simulink model "Laengsdynamikmodell_NEmo_MonteCarlo"  (R2019b)
settings: Solver=FixedStepAuto  StartTime=0.0  StopTime=1  FixedStep=SampleTime  RelTol=1e-3
undefined symbols (not defined in the file): C_RR, DiscIntNeverNeededParam, gravity, OM_PEl_M_Map, omega_Mot, PEl_MotVector, power_map_Mot, r_dyn, torque_Mot, UncertaintyMappedLosses, UncertaintyRollerDynamometer, UncertaintyTabledConsumption, VehMass
libraries: Driver_PI x1, Longitudinal_DrivingCycles x1, Acceleration_Calculation x1, Air_Resistance x1, Roll_Resistance x1, Slope_Resistance x1, Simple_Auxiliary x1, Gear_Stage x1, DCAC_Converter x1
(part 1 of 2)
settings Model: SimulationMode=accelerator  NumberOfSteps=1000  OrderedModelArguments=off  Creator=Tony  LastModifiedBy=ga69qig
settings DataIOCC: ReturnWorkspaceOutputs=off
settings DebuggingCC: ArithmeticOperatorsInVariantConditions=warning
settings SFSimCC: SimUseLocalCustomCode=off  CustomCodeUndefinedFunction=UseInterfaceOnly
settings RTWCC: RTWUseLocalCustomCode=off
settings CodeAppCC: StateflowObjectComments=on

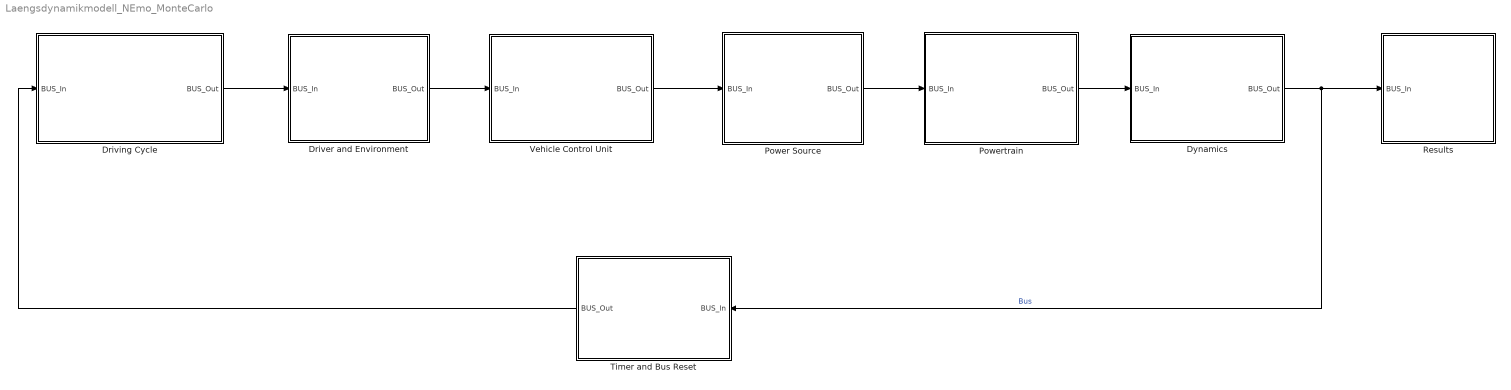
== system Laengsdynamikmodell_NEmo_MonteCarlo ==
  Driver and Environment : Subsystem
      mask help:
      | <Author> Alexander Koch based on Stefan Müller, Stephan Rohr
      | <Date> 03/04/2017
      |
      | <Description>
      | Consist of a Bus In and a Bus Out Block. To Select Signals from the Bus open the Bus In Block, to write signals to the Bus under a certain tab name open the bus out block. For further information, please read the discription of the Bus In and Bus out Block
      |
      | The Block automaticlly disconnects the link to the library block after opening the first time
      |
      | <Parameters>
      | -
      |
      | <Inputs>
      | BUS_In [Bus]
      |
      | <Outputs>
      | Bus_Out [Bus]
      settings: OpenFcn=|
      | set_param(gcb(),'LinkStatus','none')
      | open_system(gcb(),'force')
      mask Display:
      | [picturexpos,pictureypos,picturewidth,pictureheight] = ...
      |     CalcBlockPicturePosition(gcb,1,0.01,0.1,30,30); % calculating picture position depending on Block size and minimum margin size
      | image('Driver_PI.svg',[picturexpos pictureypos picturewidth pictureheight]); % plot picture to block
  Driving Cycle : Subsystem
      mask help:
      | <Author> Alexander Koch based on Stefan Müller, Stephan Rohr
      | <Date> 03/04/2017
      |
      | <Description>
      | Consist of a Bus In and a Bus Out Block. To Select Signals from the Bus open the Bus In Block, to write signals to the Bus under a certain tab name open the bus out block. For further information, please read the discription of the Bus In and Bus out Block
      |
      | The Block automaticlly disconnects the link to the library block after opening the first time
      |
      | <Parameters>
      | -
      |
      | <Inputs>
      | BUS_In [Bus]
      |
      | <Outputs>
      | Bus_Out [Bus]
      settings: OpenFcn=|
      | set_param(gcb(),'LinkStatus','none')
      | open_system(gcb(),'force')
      mask Display:
      | [picturexpos,pictureypos,picturewidth,pictureheight] = ...
      |     CalcBlockPicturePosition(gcb,1,0.01,0.1,50,50); % calculating picture position depending on Block size and minimum margin size
      | image('Longitudinal_DrivingCycles.svg',[picturexpos pictureypos picturewidth pictureheight]); % plot picture to block
  Dynamics : Subsystem
      mask help:
      | <Author> Alexander Koch based on Stefan Müller, Stephan Rohr
      | <Date> 03/04/2017
      |
      | <Description>
      | Consist of a Bus In and a Bus Out Block. To Select Signals from the Bus open the Bus In Block, to write signals to the Bus under a certain tab name open the bus out block. For further information, please read the discription of the Bus In and Bus out Block
      |
      | The Block automaticlly disconnects the link to the library block after opening the first time
      |
      | <Parameters>
      | -
      |
      | <Inputs>
      | BUS_In [Bus]
      |
      | <Outputs>
      | Bus_Out [Bus]
      settings: OpenFcn=|
      | set_param(gcb(),'LinkStatus','none')
      | open_system(gcb(),'force')
      mask Display:
      | [picturexpos,pictureypos,picturewidth,pictureheight] = ...
      |     CalcBlockPicturePosition(gcb,1,0.01,0.1,40,50); % calculating picture position depending on Block size and minimum margin size
      | image('Acceleration_Calculation.svg',[picturexpos pictureypos picturewidth pictureheight]); % plot picture to block
  Power Source : Subsystem
      mask help:
      | <Author> Alexander Koch based on Stefan Müller, Stephan Rohr
      | <Date> 03/04/2017
      |
      | <Description>
      | Consist of a Bus In and a Bus Out Block. To Select Signals from the Bus open the Bus In Block, to write signals to the Bus under a certain tab name open the bus out block. For further information, please read the discription of the Bus In and Bus out Block
      |
      | The Block automaticlly disconnects the link to the library block after opening the first time
      |
      | <Parameters>
      | -
      |
      | <Inputs>
      | BUS_In [Bus]
      |
      | <Outputs>
      | Bus_Out [Bus]
      settings: OpenFcn=|
      | set_param(gcb(),'LinkStatus','none')
      | open_system(gcb(),'force')
      mask Display:
      | [picturexpos,pictureypos,picturewidth,pictureheight] = ...
      |     CalcBlockPicturePosition(gcb,3/6,0.01,0.1,40,40); % calculating picture position depending on Block size and minimum margin size
      | image('Constant_Power_Source.svg',[picturexpos pictureypos picturewidth pictureheight]); % plot picture to block
  Powertrain : Subsystem
      mask help:
      | <Author> Alexander Koch based on Stefan Müller, Stephan Rohr
      | <Date> 03/04/2017
      |
      | <Description>
      | Consist of a Bus In and a Bus Out Block. To Select Signals from the Bus open the Bus In Block, to write signals to the Bus under a certain tab name open the bus out block. For further information, please read the discription of the Bus In and Bus out Block
      |
      | The Block automaticlly disconnects the link to the library block after opening the first time
      |
      | <Parameters>
      | -
      |
      | <Inputs>
      | BUS_In [Bus]
      |
      | <Outputs>
      | Bus_Out [Bus]
      settings: OpenFcn=|
      | set_param(gcb(),'LinkStatus','none')
      | open_system(gcb(),'force')
      mask Display:
      | [picturexpos,pictureypos,picturewidth,pictureheight] = ...
      |     CalcBlockPicturePosition(gcb,1,0.01,0.1,40,40); % calculating picture position depending on Block size and minimum margin size
      | image('Electric_Drive_Simple_Efficiency.svg',[picturexpos pictureypos picturewidth pictureheight]); % plot picture to block
  Results : Subsystem
      mask help:
      | <Author> Alexander Koch
      | <Date> 03/04/2017
      | <Predecessor> Stefan Müller, Stephan Rohr
      |
      | <Description>
      | Consist of a Bus In and a Bus Out Block. To Select Signals from the Bus open the Bus In Block, to write signals to the Bus under a certain tab name open the bus out block. For further information, please read the discription of the Bus In and Bus out Block
      |
      | The Block automaticlly disconnects the link to the library block after opening the first time
      |
      | <Parameters>
      | -
      |
      | <Inputs>
      | Bus [Bus]
      |
      | <Outputs>
      | Bus [Bus]
      settings: OpenFcn=|
      | set_param(gcb(),'LinkStatus','none')
      | open_system(gcb(),'force')
      mask Display:
      | [picturexpos,pictureypos,picturewidth,pictureheight] = ...
      |     CalcBlockPicturePosition(gcb,1,0.01,0.1,40,10); % calculating picture position depending on Block size and minimum margin size
      | image('Scopes_Simulation.svg',[picturexpos pictureypos picturewidth pictureheight]); % plot picture to block
  Timer and Bus Reset : Subsystem
      settings: OpenFcn=|
      | set_param(gcb(),'LinkStatus','none')
      | open_system(gcb(),'mask')
      mask DialogControl RefreshBus Prompt: Refresh Bus
      mask DialogControl RefreshBus Callback: TimerandBusResetRefreshBus()
      mask Display:
      | [picturexpos,pictureypos,picturewidth,pictureheight] = ...
      |     CalcBlockPicturePosition(gcb,1,0.01,0.1,50,50); % calculating picture position depending on Block size and minimum margin size
      | image('reset.png',[picturexpos pictureypos picturewidth pictureheight]); % plot picture to block
  Vehicle Control Unit : Subsystem
      mask help:
      | <Author> Alexander Koch based on Stefan Müller, Stephan Rohr
      | <Date> 03/04/2017
      |
      | <Description>
      | Consist of a Bus In and a Bus Out Block. To Select Signals from the Bus open the Bus In Block, to write signals to the Bus under a certain tab name open the bus out block. For further information, please read the discription of the Bus In and Bus out Block
      |
      | The Block automaticlly disconnects the link to the library block after opening the first time
      |
      | <Parameters>
      | -
      |
      | <Inputs>
      | BUS_In [Bus]
      |
      | <Outputs>
      | Bus_Out [Bus]
      settings: OpenFcn=|
      | set_param(gcb(),'LinkStatus','none')
      | open_system(gcb(),'force')
      mask Display:
      | [picturexpos,pictureypos,picturewidth,pictureheight] = ...
      |     CalcBlockPicturePosition(gcb,1,0.01,0.1,30,30); % calculating picture position depending on Block size and minimum margin size
      | image('Control_Unit_Simple.svg',[picturexpos pictureypos picturewidth pictureheight]); % plot picture to block
  wires:
  Power Source/1(BUS_Out) -> Powertrain/1(BUS_In)
  Driver and Environment/1(BUS_Out) -> Vehicle Control Unit/1(BUS_In)
  Driving Cycle/1(BUS_Out) -> Driver and Environment/1(BUS_In)
  Vehicle Control Unit/1(BUS_Out) -> Power Source/1(BUS_In)
  Timer and Bus Reset/1(BUS_Out) -> Driving Cycle/1(BUS_In)
  Dynamics/1(BUS_Out) -> Timer and Bus Reset/1(BUS_In), Results/1(BUS_In)  "Bus"
  Powertrain/1(BUS_Out) -> Dynamics/1(BUS_In)

== system Laengsdynamikmodell_NEmo_MonteCarlo/Driver and Environment ==
  BUS_In : Inport
  BUS IN : Subsystem
      mask help:
      | <Author> Alexander Koch based on Stefan Müller, Stephan Rohr
      | <Date> 02/05/2017
      |
      | <Description>
      | Automated BUS IN Block for the Bus System. After the Bus In is connected and receives signals it is possible to choose the required signals by clicking on the block. After choosing the signals it is possible to push the Refresh button. This button builds the required amount of outputs, connects the Bus Selector and the Outputs and rename all the outputs with the corresponding signal name.
      |
      | The Block automaticlly disconnects the link to the library block after opening the first time
      |
      | <Parameters>
      | -
      |
      | <Inputs>
      | Bus [Bus]
      |
      | <Outputs>
      | Bus [Bus]
      | SignalName[-]
      mask init:
      | BusInInitFct()
      settings: OpenFcn=|
      | set_param(gcb(),'LinkStatus','none')
      | open_system(gcb(),'mask')
      | open_system(strcat(gcb(),'/Bus Selector'),'Parameter')
      mask DialogControl ParameterGroupVar Prompt: Refresh
      mask DialogControl RefreshOutputs Prompt: Refresh all Output Names
      mask DialogControl RefreshOutputs Callback: BusInInitFct()
  BUS OUT : Subsystem  mask{NumberofInputs=6, NameSys='Driver and Enironment'}
      mask prompts: NumberofInputs "Numper of costum inputs"; NameSys "Name of Bus Subsystem"
      mask help:
      | <Author> Alexander Koch based on Stefan Müller, Stephan Rohr
      | <Date> 02/05/2017
      |
      | <Description>
      | Automated BUS Out Block for the Bus System. Allows to enter the Number of costum inputs and the name of the bus system. After entering the parameters the required amout of Inputs are built and connected to the Bus Creator. The signal names that are connected to the inputs In1, ..., InN are automatically adopted at the Bus signal names and can be found in the Bus under the name of the Bus Subsystem. If the signal (line) to the Inport has no name, the name of the previous blocks outport is taken. If this is not possible, the name if the previous block is taken for the Bus signal name.
      |
      | Additional, there are two buttons. The Refresh Input Names refreshes all Input Names. This is required if signal names are changed or signals are connected for the first time. To build a new system or if another Subsystem is added between existing subsystems, the Refresh Bus Selector is required at every subsystem that is calculated after the new subsystem.
      |
      | The Block automaticlly disconnects the link to the library block after opening the first time
      |
      | <Parameters>
      | Number of costum inputs [-]
      | Name of Bus Subsystem ['abc']
      |
      | <Inputs>
      | Bus [Bus]
      | In1 [ ]
      |
      | <Outputs>
      | Bus [Bus]
      mask init:
      | BusRefreshInputs()
      settings: OpenFcn=|
      | set_param(gcb(),'LinkStatus','none')
      | open_system(gcb(),'mask')
      mask DialogControl Container3 Prompt: Refresh
      mask DialogControl RefreshInputNames Prompt: Refresh Input Names
      mask DialogControl RefreshInputNames Callback: BusRefreshLineNames()
      mask DialogControl RefreshBusSelector Prompt: Refresh Bus Selector
      mask DialogControl RefreshBusSelector Callback: BusRefreshBusSelector()
  Constant Environment : Subsystem  AncestorBlock=Constant_Environment/Constant Environment  mask(SB){Ground_Slope=0, Long_Wind_Speed=0, Ambient_P=101325, Ambient_Temp=293.15, LocalSampleTime=-1}
      mask prompts: Ground_Slope "Ground Slope [rad]"; Long_Wind_Speed "Longitudinal Wind Velocity [m/s]"; Ambient_P "Ambient Pressure [Pa]"; Ambient_Temp "Ambient Temperature [K]"; LocalSampleTime "Local System Sample-Time [s]"
      mask help:
      | <Author> Tony Weiss based on Alexander Koch </Author>
      | <Date> 31/12/2017 </Date>
      | <Source>
      | [1] A. Koch, “Aufbau einer modularen Komponentenbibliothek für Gesamtfahrzeugsimulationen in Matlab/Simulink,” Technische Universität München, München, 2017
      | </Source>
      |
      | <Description>
      | Requires a ground slope, a longitudinal wind velocity, an ambient temperature and an ambient pressure and gives these constant values as signals. Ambient pressure is preset to 101325 Pa (standard pressure at sea level), ambient temperature is preset to 298.15 K.
      | </Description>
      mask init:
      | GlobalSampleTime = CalcGlobalSampleTime(LocalSampleTime);
      mask Help:
      | <Parameters>
      | Ground Slope [rad]
      | Longitudinal Wind Velocity [m/s]
      | Ambient Temperature [K]
      | Ambient Pressure [Pa]
      | Local System Sample-Time [s]
      | 	<Min> GlobalSampleTime </Min>
      | Global Sample-Time [s]
      | </Parameters>
      | 
      | <Inputs>
      | </Inputs>
      | 
      | <Outputs>
      | GroundSlope [rad]
      | LongWindVelocity [m/s]
      | AmbientTemperature [K]
      | AmbientPressure [Pa]
      | </Outputs>
      mask TypeOptions Ground_Slope: Const_Ground_Slope/Value
      mask TypeOptions Long_Wind_Speed: Const_Long_Wind_Velocity/Value
      mask TypeOptions Ambient_P: Const_Ambient_Pressure/Value
      mask TypeOptions Ambient_Temp: Const_Ambient_Temperature/Value
      mask TypeOptions LocalSampleTime: Const_Ambient_Pressure/SampleTime | Const_Ambient_Temperature/SampleTime | Const_Ground_Slope/SampleTime | Const_Long_Wind_Velocity/SampleTime
      mask DialogControl Container3 Prompt: Documentation:
      mask DialogControl Control2 Prompt: %<MaskHelp>
      mask DialogControl Container5 Prompt: Sample Time
      mask Display:
      | [picturexpos,pictureypos,picturewidth,pictureheight] = ...
      |     CalcBlockPicturePosition(gcb,1,0.01,0.1,10,100); % calculating picture position depending on Block size and minimum margin size
      | image('Constant_Environment.svg',[picturexpos pictureypos picturewidth pictureheight]) % plot picture to block
  Driver PI : Driver_PI/Driver PI  ThrottleP=7  ThrottleI=1  BrakeP=7  BrakeI=1.5  WeightingFactorPrecontrol=0  MaxVehicleSpeed=80  hysteresis=0.05  LocalSampleTime=-1
  BUS_Out : Outport  VectorParamsAs1DForOutWhenUnconnected=off
  wires:
  BUS IN/1(BUS) -> BUS OUT/1(BUS)
  BUS OUT/1(BUS_OUT) -> BUS_Out/1
  BUS_In/1 -> BUS IN/1(BUS_In)
  BUS IN/2(v [m/s]) -> Driver PI/1
  Driver PI/1 -> BUS OUT/2(In1)
  Driver PI/2 -> BUS OUT/3(In2)
  Constant Environment/1(GroundSlope [rad]) -> BUS OUT/4(In3)
  Constant Environment/2(LongWindVelocity [m/s]) -> BUS OUT/5(In4)
  BUS IN/3(VehSpd [m/s]) -> Driver PI/2
  Constant Environment/3(AmbientTemperature [K]) -> BUS OUT/6(In5)
  Constant Environment/4(AmbientPressure [Pa]) -> BUS OUT/7(In6)

== system Laengsdynamikmodell_NEmo_MonteCarlo/Driving Cycle ==
  BUS_In : Inport
  BUS IN : Subsystem
      mask help:
      | <Author> Alexander Koch
      | <Date> 02/05/2017
      | <Predecessor> Stefan Müller, Stephan Rohr
      |
      | <Description>
      | Automated BUS IN Block for the Bus System. After the Bus In is connected and receives signals it is possible to choose the required signals by clicking on the block. After choosing the signals it is possible to push the Refresh button. This button builds the required amount of outputs, connects the Bus Selector and the Outputs and rename all the outputs with the corresponding signal name.
      |
      | The Block automaticlly disconnects the link to the library block after opening the first time
      |
      | <Parameters>
      | -
      |
      | <Inputs>
      | Bus [Bus]
      |
      | <Outputs>
      | Bus [Bus]
      | SignalName[-]
      mask init:
      | BusInInitFct()
      settings: OpenFcn=|
      | set_param(gcb(),'LinkStatus','none')
      | open_system(gcb(),'mask')
      | open_system(strcat(gcb(),'/Bus Selector'),'Parameter')
      mask DialogControl ParameterGroupVar Prompt: Refresh
      mask DialogControl RefreshOutputs Prompt: Refresh all Output Names
      mask DialogControl RefreshOutputs Callback: BusInInitFct()
  BUS OUT : Subsystem  mask{NumberofInputs=4, NameSys='DrivinCycle'}
      mask prompts: NumberofInputs "Numper of costum inputs"; NameSys "Name of Bus Subsystem"
      mask help:
      | <Author> Alexander Koch based on Stefan Müller, Stephan Rohr
      | <Date> 02/05/2017
      |
      | <Description>
      | Automated BUS Out Block for the Bus System. Allows to enter the Number of costum inputs and the name of the bus system. After entering the parameters the required amout of Inputs are built and connected to the Bus Creator. The signal names that are connected to the inputs In1, ..., InN are automatically adopted at the Bus signal names and can be found in the Bus under the name of the Bus Subsystem. If the signal (line) to the Inport has no name, the name of the previous blocks outport is taken. If this is not possible, the name if the previous block is taken for the Bus signal name.
      |
      | Additional, there are two buttons. The Refresh Input Names refreshes all Input Names. This is required if signal names are changed or signals are connected for the first time. To build a new system or if another Subsystem is added between existing subsystems, the Refresh Bus Selector is required at every subsystem that is calculated after the new subsystem.
      |
      | The Block automaticlly disconnects the link to the library block after opening the first time
      |
      | <Parameters>
      | Number of costum inputs [-]
      | Name of Bus Subsystem ['abc']
      |
      | <Inputs>
      | Bus [Bus]
      | In1 [ ]
      |
      | <Outputs>
      | Bus [Bus]
      mask init:
      | BusRefreshInputs()
      settings: OpenFcn=|
      | set_param(gcb(),'LinkStatus','none')
      | open_system(gcb(),'mask')
      mask DialogControl Container3 Prompt: Refresh
      mask DialogControl RefreshInputNames Prompt: Refresh Input Names
      mask DialogControl RefreshInputNames Callback: BusRefreshLineNames()
      mask DialogControl RefreshBusSelector Prompt: Refresh Bus Selector
      mask DialogControl RefreshBusSelector Callback: BusRefreshBusSelector()
  Longitudinal Driving Cycles : Longitudinal_DrivingCycles/Longitudinal Driving Cycles  dcname=Custom_Driving_Cycle  dccircuits=1  dc_speed=cycle  dc_gear=[]  LocalSampleTime=-1
  Terminator : Terminator
  BUS_Out : Outport  VectorParamsAs1DForOutWhenUnconnected=off
  wires:
  BUS IN/1(BUS) -> BUS OUT/1(BUS)
  BUS OUT/1(BUS_OUT) -> BUS_Out/1
  BUS_In/1 -> BUS IN/1(BUS_In)
  Longitudinal Driving Cycles/1 -> BUS OUT/2(In1)  "v [m/s]"
  Longitudinal Driving Cycles/2 -> BUS OUT/3(In2)
  Longitudinal Driving Cycles/3 -> BUS OUT/4(In3)
  Longitudinal Driving Cycles/4 -> BUS OUT/5(In4)
  BUS IN/2(VehSpd [m/s]) -> Terminator/1

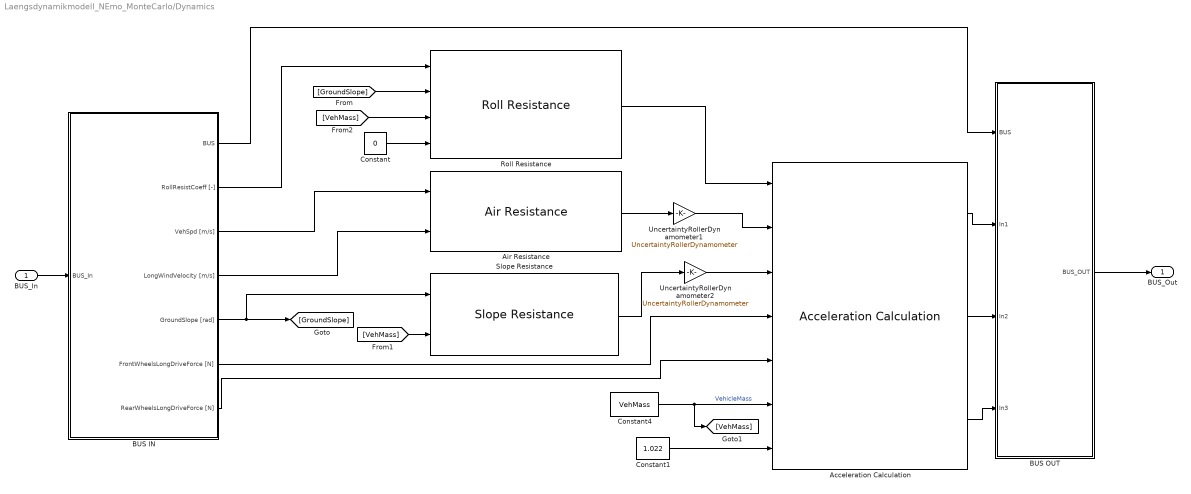
== system Laengsdynamikmodell_NEmo_MonteCarlo/Dynamics ==
  BUS_In : Inport
  Acceleration Calculation : Acceleration_Calculation/Acceleration Calculation  InitialCondition=0  LocalSampleTime=-1
  Air Resistance : Air_Resistance/Air Resistance  A_st=1.947  Roh_Air=rho_L  c_w=0.37  LocalSampleTime=-1
  BUS IN : Subsystem
      mask help:
      | <Author> Alexander Koch
      | <Date> 02/05/2017
      | <Predecessor> Stefan Müller, Stephan Rohr
      |
      | <Description>
      | Automated BUS IN Block for the Bus System. After the Bus In is connected and receives signals it is possible to choose the required signals by clicking on the block. After choosing the signals it is possible to push the Refresh button. This button builds the required amount of outputs, connects the Bus Selector and the Outputs and rename all the outputs with the corresponding signal name.
      |
      | The Block automaticlly disconnects the link to the library block after opening the first time
      |
      | <Parameters>
      | -
      |
      | <Inputs>
      | Bus [Bus]
      |
      | <Outputs>
      | Bus [Bus]
      | SignalName[-]
      mask init:
      | BusInInitFct()
      settings: OpenFcn=|
      | set_param(gcb(),'LinkStatus','none')
      | open_system(gcb(),'mask')
      | open_system(strcat(gcb(),'/Bus Selector'),'Parameter')
      mask DialogControl ParameterGroupVar Prompt: Refresh
      mask DialogControl RefreshOutputs Prompt: Refresh all Output Names
      mask DialogControl RefreshOutputs Callback: BusInInitFct()
  BUS OUT : Subsystem  mask{NumberofInputs=3, NameSys='Dynamics'}
      mask prompts: NumberofInputs "Numper of costum inputs"; NameSys "Name of Bus Subsystem"
      mask help:
      | <Author> Alexander Koch
      | <Date> 02/05/2017
      | <Predecessor> Stefan Müller, Stephan Rohr
      |
      | <Description>
      | Automated BUS Out Block for the Bus System. Allows to enter the Number of costum inputs and the name of the bus system. After entering the parameters the required amout of Inputs are built and connected to the Bus Creator. The signal names that are connected to the inputs In1, ..., InN are automatically adopted at the Bus signal names and can be found in the Bus under the name of the Bus Subsystem. If the signal (line) to the Inport has no name, the name of the previous blocks outport is taken. If this is not possible, the name if the previous block is taken for the Bus signal name.
      |
      | Additional, there are two buttons. The Refresh Input Names refreshes all Input Names. This is required if signal names are changed or signals are connected for the first time. To build a new system or if another Subsystem is added between existing subsystems, the Refresh Bus Selector is required at every subsystem that is calculated after the new subsystem.
      |
      | The Block automaticlly disconnects the link to the library block after opening the first time
      |
      | <Parameters>
      | Number of costum inputs [-]
      | Name of Bus Subsystem ['abc']
      |
      | <Inputs>
      | Bus [Bus]
      | In1 [ ]
      |
      | <Outputs>
      | Bus [Bus]
      mask init:
      | BusRefreshInputs()
      settings: OpenFcn=|
      | set_param(gcb(),'LinkStatus','none')
      | open_system(gcb(),'mask')
      mask DialogControl Container3 Prompt: Refresh
      mask DialogControl RefreshInputNames Prompt: Refresh Input Names
      mask DialogControl RefreshInputNames Callback: BusRefreshLineNames()
      mask DialogControl RefreshBusSelector Prompt: Refresh Bus Selector
      mask DialogControl RefreshBusSelector Callback: BusRefreshBusSelector()
  Constant : Constant  Value=0
  Constant1 : Constant  Value=1.022
  Constant4 : Constant  Value=VehMass  SampleTime=-1
  Roll Resistance : Roll_Resistance/Roll Resistance  Gravity=gravity  LocalSampleTime=-1
  Slope Resistance : Slope_Resistance/Slope Resistance  Gravity=gravity  LocalSampleTime=-1
  UncertaintyRollerDynamometer1 : Gain  Gain=UncertaintyRollerDynamometer
  UncertaintyRollerDynamometer2 : Gain  Gain=UncertaintyRollerDynamometer
  BUS_Out : Outport  VectorParamsAs1DForOutWhenUnconnected=off
  wires:
  BUS IN/1(BUS) -> BUS OUT/1(BUS)
  BUS OUT/1(BUS_OUT) -> BUS_Out/1
  BUS_In/1 -> BUS IN/1(BUS_In)
  BUS IN/2(RollResistCoeff [-]) -> Roll Resistance/1
  BUS IN/4(LongWindVelocity [m/s]) -> Air Resistance/2
  [GroundSlope] -> Roll Resistance/2
  BUS IN/5(GroundSlope [rad]) -> Slope Resistance/1, [GroundSlope]
  Air Resistance/1 -> UncertaintyRollerDynamometer1/1
  Slope Resistance/1 -> UncertaintyRollerDynamometer2/1
  BUS IN/6(FrontWheelsLongDriveForce [N]) -> Acceleration Calculation/4
  BUS IN/7(RearWheelsLongDriveForce [N]) -> Acceleration Calculation/5
  Constant4/1 -> [VehMass], Acceleration Calculation/6  "VehicleMass"
  [VehMass] -> Slope Resistance/2
  [VehMass] -> Roll Resistance/3
  Constant/1 -> Roll Resistance/4
  Constant1/1 -> Acceleration Calculation/7
  Acceleration Calculation/1 -> BUS OUT/2(In1)
  Acceleration Calculation/2 -> BUS OUT/3(In2)
  Acceleration Calculation/3 -> BUS OUT/4(In3)
  BUS IN/3(VehSpd [m/s]) -> Air Resistance/1
  Roll Resistance/1 -> Acceleration Calculation/1
  UncertaintyRollerDynamometer1/1 -> Acceleration Calculation/2
  UncertaintyRollerDynamometer2/1 -> Acceleration Calculation/3

== system Laengsdynamikmodell_NEmo_MonteCarlo/Power Source ==
  note: During the experiments the vehicle Smart Fortwo
      | was pluged in to a battery simulator, which provides
      | a power source with constant voltage.
  BUS_In : Inport
  Add : Sum
  BUS IN : Subsystem
      mask help:
      | <Author> Alexander Koch based on Stefan Müller, Stephan Rohr
      | <Date> 02/05/2017
      |
      | <Description>
      | Automated BUS IN Block for the Bus System. After the Bus In is connected and receives signals it is possible to choose the required signals by clicking on the block. After choosing the signals it is possible to push the Refresh button. This button builds the required amount of outputs, connects the Bus Selector and the Outputs and rename all the outputs with the corresponding signal name.
      |
      | The Block automaticlly disconnects the link to the library block after opening the first time
      |
      | <Parameters>
      | -
      |
      | <Inputs>
      | Bus [Bus]
      |
      | <Outputs>
      | Bus [Bus]
      | SignalName[-]
      mask init:
      | BusInInitFct()
      settings: OpenFcn=|
      | set_param(gcb(),'LinkStatus','none')
      | open_system(gcb(),'mask')
      | open_system(strcat(gcb(),'/Bus Selector'),'Parameter')
      mask DialogControl ParameterGroupVar Prompt: Refresh
      mask DialogControl RefreshOutputs Prompt: Refresh all Output Names
      mask DialogControl RefreshOutputs Callback: BusInInitFct()
  BUS OUT : Subsystem  mask{NumberofInputs=3, NameSys='Powersource'}
      mask prompts: NumberofInputs "Numper of costum inputs"; NameSys "Name of Bus Subsystem"
      mask help:
      | <Author> Alexander Koch based on Stefan Müller, Stephan Rohr
      | <Date> 02/05/2017
      |
      | <Description>
      | Automated BUS Out Block for the Bus System. Allows to enter the Number of costum inputs and the name of the bus system. After entering the parameters the required amout of Inputs are built and connected to the Bus Creator. The signal names that are connected to the inputs In1, ..., InN are automatically adopted at the Bus signal names and can be found in the Bus under the name of the Bus Subsystem. If the signal (line) to the Inport has no name, the name of the previous blocks outport is taken. If this is not possible, the name if the previous block is taken for the Bus signal name.
      |
      | Additional, there are two buttons. The Refresh Input Names refreshes all Input Names. This is required if signal names are changed or signals are connected for the first time. To build a new system or if another Subsystem is added between existing subsystems, the Refresh Bus Selector is required at every subsystem that is calculated after the new subsystem.
      |
      | The Block automaticlly disconnects the link to the library block after opening the first time
      |
      | <Parameters>
      | Number of costum inputs [-]
      | Name of Bus Subsystem ['abc']
      |
      | <Inputs>
      | Bus [Bus]
      | In1 [ ]
      |
      | <Outputs>
      | Bus [Bus]
      mask init:
      | BusRefreshInputs()
      settings: OpenFcn=|
      | set_param(gcb(),'LinkStatus','none')
      | open_system(gcb(),'mask')
      mask DialogControl Container3 Prompt: Refresh
      mask DialogControl RefreshInputNames Prompt: Refresh Input Names
      mask DialogControl RefreshInputNames Callback: BusRefreshLineNames()
      mask DialogControl RefreshBusSelector Prompt: Refresh Bus Selector
      mask DialogControl RefreshBusSelector Callback: BusRefreshBusSelector()
  Constant Power Source : Subsystem  mask(SB){MaxPower=400000, MinPower=-10000}
      mask prompts: MaxPower "Maximum Power [W]"; MinPower "Minimum Power [W]"
      mask help:
      | <Author> Tony Weiss based on Nikolaos Wassiliadis, Michael Baumann </Author>
      | <Date> 22/04/2018 </Date>
      |
      | <Description>
      | Inside this battery model is the battery cell Panasonic 18650PF which calculates all cell parameters. Through the number of cells parallel and serial, the battery power and voltage is calculated. The model therefore needs the initals values of SOC, U_RC1 and U_RC2 of the cell.
      | </Description>
      mask Help:
      | <Parameters>
      | Cells Serial [-]
      | 	<Min> 1 </Min>
      | Cells Parallel [-]
      | 	<Min> 1 </Min>
      | Initial Cell State [3x1]
      | 	--> [SOC;U_RC1;U_RC2]
      | 
      | 	SOC: 	<Min> 0 </Min>
      | 		<Max> 1 </Max>
      | 	U_RC1:	<Min> 0 </Min>
      | 	U_RC2:	<Min> 0 </Min>
      | </Parameters>
      | 
      | <Inputs>
      | CellPara_x_k [-]
      | 	3x1 Vector --> [SOC;U_RC1;U_RC2]
      | CellVoltage_x_k [V]
      | BatPowerReq [W]
      | 	<sign orientation> [+] discharge </sign orientation>
      | </Inputs>
      | 
      | <Outputs>
      | SOC [-]
      | 	<Min> 0 </Min>
      | 	<Max> 1 </Max>
      | CellPara_x_k+1 [-]
      | 	3x1 Vector --> [SOC;U_RC1;U_RC2]
      | CellVoltage_x_k+1 [V]
      | BatPowerAvl [W]
      | 	<sign orientation> [+] discharge </sign orientation>
      | </Outputs>
      mask DialogControl Container3 Prompt: Documentation:
      mask DialogControl Control2 Prompt: %<MaskHelp>
  Simple Auxiliary : Simple_Auxiliary/Simple Auxiliary  AuxPower=142.6  LocalSampleTime=0
  BUS_Out : Outport  VectorParamsAs1DForOutWhenUnconnected=off
  wires:
  BUS IN/1(BUS) -> BUS OUT/1(BUS)
  BUS OUT/1(BUS_OUT) -> BUS_Out/1
  BUS_In/1 -> BUS IN/1(BUS_In)
  Constant Power Source/1(ActualPower [W]) -> BUS OUT/2(In1)
  Constant Power Source/2(MaxPower [W]) -> BUS OUT/3(In2)
  Constant Power Source/3(MinPower [W]) -> BUS OUT/4(In3)
  BUS IN/2(PowertrainPowerReq [W]) -> Add/2
  Add/1 -> Constant Power Source/1(RequiredPower [W])
  Simple Auxiliary/1 -> Add/1  "AuxiliariesPower [W]"

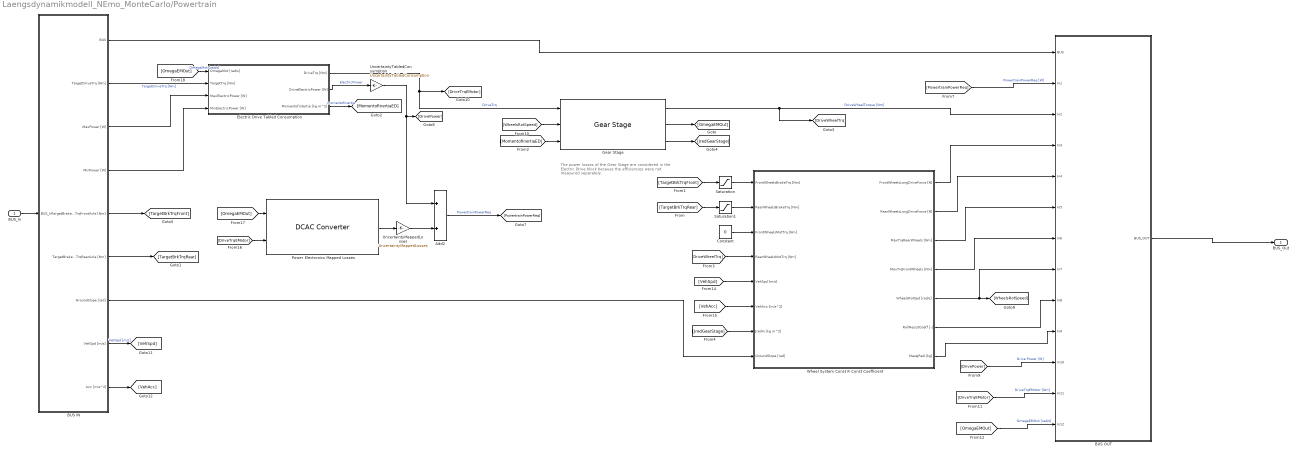
== system Laengsdynamikmodell_NEmo_MonteCarlo/Powertrain ==
  note: The power losses of the Gear Stage are considered
      | in the Electric Drive block because the efficiencies were
      | not measured separately.
  BUS_In : Inport
  Add2 : Sum
  BUS IN : Subsystem
      mask help:
      | <Author> Alexander Koch based on Stefan Müller, Stephan Rohr
      | <Date> 02/05/2017
      |
      | <Description>
      | Automated BUS IN Block for the Bus System. After the Bus In is connected and receives signals it is possible to choose the required signals by clicking on the block. After choosing the signals it is possible to push the Refresh button. This button builds the required amount of outputs, connects the Bus Selector and the Outputs and rename all the outputs with the corresponding signal name.
      |
      | The Block automaticlly disconnects the link to the library block after opening the first time
      |
      | <Parameters>
      | -
      |
      | <Inputs>
      | Bus [Bus]
      |
      | <Outputs>
      | Bus [Bus]
      | SignalName[-]
      mask init:
      | BusInInitFct()
      settings: OpenFcn=|
      | set_param(gcb(),'LinkStatus','none')
      | open_system(gcb(),'mask')
      | open_system(strcat(gcb(),'/Bus Selector'),'Parameter')
      mask DialogControl ParameterGroupVar Prompt: Refresh
      mask DialogControl RefreshOutputs Prompt: Refresh all Output Names
      mask DialogControl RefreshOutputs Callback: BusInInitFct()
  BUS OUT : Subsystem  mask{NumberofInputs=12, NameSys='Powertrain'}
      mask prompts: NumberofInputs "Numper of costum inputs"; NameSys "Name of Bus Subsystem"
      mask help:
      | <Author> Alexander Koch based on Stefan Müller, Stephan Rohr
      | <Date> 02/05/2017
      |
      | <Description>
      | Automated BUS Out Block for the Bus System. Allows to enter the Number of costum inputs and the name of the bus system. After entering the parameters the required amout of Inputs are built and connected to the Bus Creator. The signal names that are connected to the inputs In1, ..., InN are automatically adopted at the Bus signal names and can be found in the Bus under the name of the Bus Subsystem. If the signal (line) to the Inport has no name, the name of the previous blocks outport is taken. If this is not possible, the name if the previous block is taken for the Bus signal name.
      |
      | Additional, there are two buttons. The Refresh Input Names refreshes all Input Names. This is required if signal names are changed or signals are connected for the first time. To build a new system or if another Subsystem is added between existing subsystems, the Refresh Bus Selector is required at every subsystem that is calculated after the new subsystem.
      |
      | The Block automaticlly disconnects the link to the library block after opening the first time
      |
      | <Parameters>
      | Number of costum inputs [-]
      | Name of Bus Subsystem ['abc']
      |
      | <Inputs>
      | Bus [Bus]
      | In1 [ ]
      |
      | <Outputs>
      | Bus [Bus]
      mask init:
      | BusRefreshInputs()
      settings: OpenFcn=|
      | set_param(gcb(),'LinkStatus','none')
      | open_system(gcb(),'mask')
      mask DialogControl Container3 Prompt: Refresh
      mask DialogControl RefreshInputNames Prompt: Refresh Input Names
      mask DialogControl RefreshInputNames Callback: BusRefreshLineNames()
      mask DialogControl RefreshBusSelector Prompt: Refresh Bus Selector
      mask DialogControl RefreshBusSelector Callback: BusRefreshBusSelector()
  Constant : Constant  Value=0
  Electric Drive Tabled Consumption : Subsystem  AncestorBlock=Electric_Drive_Tabled_Consumption/Electric Drive Tabled Consumption  mask(SB){inertia=0.03, mass=1, OM_M_Pel_Map=power_map_Mot, M_MotVector=torque_Mot, OM_MotVector=omega_Mot, M_Full_Load=[128 128 128 127 127 126 126 126 126 124 119 114 109 103 100 94 89 85 79 75 70 68 67 65 63 62 60 58 59 60 62 63 63 62 61 60 58 57 55 53 51 50 48 46 45 43 42 40 39 38 36 35 34 32 31 30 29 28 26 25 24], OM_Full_Load=[0 11.4144533080429 22.8289066160858 34.2433599241288 45.6578132321717 57.1769862953342 68.5914396033771 80.0058929114201 91.4203462194630 102.834799527506 114.249252835549 125.663706143592 137.078159451635 148.492612759678 160.011785822840 171.426239130883 182.840692438926 194.255145746969 205.669599055012 217.084052363055 228.498505671098 239.912958979141 251.327412287183 262.846585350346 274.261038658389 285.675491966432 297.089945274475 308.504398582518 319.918851890561 331.333305198604 342.747758506646 354.162211814689 365.681384877852 377.095838185895 388.510291493938 399.924744801981 411.339198110024 422.753651418066 434.168104726109 445.582558034152 456.997011342195 468.516184405358 479.930637713401 491.345091021444 502.759544329487 514.173997637529 525.588450945572 537.002904253615 548.417357561658 559.831810869701 571.350983932864 582.765437240907 594.179890548950 605.594343856992 617.008797165035 628.423250473078 639.837703781121 651.252157089164 662.666610397207 674.185783460370 685.600236768413], M_Min_Load=[0 0 0 0 0 0 0 0 0 0 0 0 0 0 0 0 0 0 0 0 0 0 0 0 0 0 0 0 0 0 0 0 0 0 0 0 0 0 0 0 0 0 0 0 0 0 0 0 0 0 0 0 0 0 0 0 0 0 0 0 0], OM_Min_Load=[0 11.4144533080429 22.8289066160858 34.2433599241288 45.6578132321717 57.1769862953342 68.5914396033771 80.0058929114201 91.4203462194630 102.834799527506 114.249252835549 125.663706143592 137.078159451635 148.492612759678 160.011785822840 171.426239130883 182.840692438926 194.255145746969 205.669599055012 217.084052363055 228.498505671098 239.912958979141 251.327412287183 262.846585350346 274.261038658389 285.675491966432 297.089945274475 308.504398582518 319.918851890561 331.333305198604 342.747758506646 354.162211814689 365.681384877852 377.095838185895 388.510291493938 399.924744801981 411.339198110024 422.753651418066 434.168104726109 445.582558034152 456.997011342195 468.516184405358 479.930637713401 491.345091021444 502.759544329487 514.173997637529 525.588450945572 537.002904253615 548.417357561658 559.831810869701 571.350983932864 582.765437240907 594.179890548950 605.594343856992 617.008797165035 628.423250473078 639.837703781121 651.252157089164 662.666610397207 674.185783460370 685.600236768413], LocalSampleTime=-1}
      mask prompts: inertia "Moment of Inertia E-Motor [kg*m^2]"; mass "Mass E-Motor [kg"; OM_M_Pel_Map "Tabled Electric Power [NxM]"; M_MotVector "Reference Torque Vector [1xM]"; OM_MotVector "Reference Omega Vector [1xN]"; M_Full_Load "Torque Vector for Full Load Line [1xL]"; OM_Full_Load "Reference Omega Vector for Full Load Line [1xL]"; M_Min_Load "Torque Vector for Min Load Line [1xK]"; OM_Min_Load "Reference Omega Vector for Min Load Line [1xK]"; LocalSampleTime "Local System Sample-Time [s]"
      mask help:
      | <Author> Benedikt Danquah based on Lorenz Horlbeck [1] and Philip Wacker [2]</Author>
      | <Date> 01/2019 </Date>
      |
      | <Description>
      | Calculates the target drive torque. The avaiable max./min. electric power of the battery limits the electric system. The mechanical system is limited by the max./min. torque curve. Due to the limits the final drive torque and the drive electric power (via 2D-Lookup table) is calculated. The moment of inertia is given as a constant signal.
      | </Description>
      mask init:
      | GlobalSampleTime = CalcGlobalSampleTime(LocalSampleTime);
      | 
      | [OM_PEl_M_Map,OM_MotVector, PEl_MotVector]= init_Electric_Drive_Tabled_Consumption (OM_M_Pel_Map,M_MotVector,OM_MotVector,M_Full_Load,OM_Full_Load,M_Min_Load,OM_Min_Load);
      | 
      | %figure
      | %hold on
      | %surfc(OM_MotVector,M_MotVector,OM_M_Pel_Map')
      | %for i=1:1000
      |  %   plot3(OM_Full_Load,M_Full_Load,ones(1,61)*i*30,'color','red', 'linewidth',6)
      | %end
      | %hold off
      | 
      | 
      | %figure
      | %surfc(OM_MotVector,PEl_Vector,OM_PEl_M_Map')
      mask Help:
      | <Parameters>
      | Moment of Inertia E-Motor [kg*m^2]
      | Mass E-Motor [kg]
      | Tabled Electric Power [NxM]
      | Reference Torque Vector [1xM]
      | Reference Omega Vector [1xN]
      | Torque Vector for Full Load Line [1xL]
      | Reference Omega Vector for Full Load Line [1xL]
      | Torque Vector for Min Load Line [1xK]
      | Reference Omega Vector for Min Load Line [1xK]
      | </Parameters>
      | 
      | with M,N,P = ∈ {ℕ}
      | 
      | <Inputs>
      | OmegaMot [rad/s]
      | TargetTrq [Nm]
      | MaxElectricPower [W]
      | 	<sign orientation> [+] discharge </sign orientation>
      | MinElectricPower  [W]
      | 	<sign orientation> [-] charge </sign orientation>
      | </Inputs>
      | 
      | <Outputs>
      | DriveTrq [Nm]
      | DriveElectricPower [W]
      | 	<sign orientation> [+] discharge </sign orientation>
      | Momentofinertia [kg*m^2]
      | </Outputs>
      | <Sources>
      | [1] L. Horlbeck, “Auslegung elektrischer Maschinen für automobile Antriebsstränge unter Berücksichtigung des Überlastpotentials,” Dissertation, Institute of Automotive Technology, Technical University Munich, Munich, 2018.
      | [2] P. Wacker, J. Adermann, B. Danquah, and M. Lienkamp, “Efficiency determination of active battery switching technology on roller dynamometer,” in Twelfth International Conference on Ecological Vehicles and Renewable Energies, Monaco, 2017, pp. 1–7.
      | </Sources>
      mask TypeOptions LocalSampleTime: OmegaMot [rad//s]/SampleTime | TargetTrq [Nm]/SampleTime | MaxElectricPower [W]/SampleTime | MinElectricPower [W]/SampleTime
      mask DialogControl Container3 Prompt: Documentation
      mask DialogControl Control4 Prompt: %<MaskHelp>
      mask DialogControl show_plot Prompt: Plot Consumption Map
      mask DialogControl show_plot Callback: PlotMaps(gcb);
      mask DialogControl Container7 Prompt: Sample Time
      mask Display:
      | [picturexpos,pictureypos,picturewidth,pictureheight] = ...
      |     CalcBlockPicturePosition(gcb,1,0.01,0.1,100,100); % calculating picture position depending on Block size and minimum margin size
      | image('Electric_Drive_Tabled_Consumption.svg',[picturexpos pictureypos picturewidth pictureheight]) % plot picture to block
  Gear Stage : Gear_Stage/Gear Stage  iGear=i_gear  eta=1  JredGetr=0.19  LocalSampleTime=-1
  Power Electronics Mapped Losses : DCAC_Converter/DCAC Converter  W_Vektor=omega_LE  M_Vektor_motgen=torque_LE  P_Loss=power_map_LE  LocalSampleTime=-1
  Saturation : Saturate  UpperLimit=0  LowerLimit=-inf
  Saturation1 : Saturate  UpperLimit=0  LowerLimit=-inf
  UncertaintyMappedLosses : Gain  Gain=UncertaintyMappedLosses
  UncertaintyTabledConsumption : Gain  Gain=UncertaintyTabledConsumption
  Wheel System Const R Const Coefficient : Subsystem  mask(SB){Wheel_Radius=r_dyn, Wheel_Roll_Resistance=C_RR, Wheel_Roll_Resistance_Dyn=0, mu_Tyre=0.7, J_FourWheels=4, Gravity=gravity, Wheelbase=1.863, COG_Height=0.5, COG_Front=1.1178, COG_Rear=0.7452, Veh_Mass=VehMass, LocalSampleTime=-1}
      mask prompts: Wheel_Radius "Wheel Radius [m]"; Wheel_Roll_Resistance "Roll Resistance Coefficient [-]"; Wheel_Roll_Resistance_Dyn "Dynamic Roll Resistance Coefficient [s/m]"; mu_Tyre "Friction Coefficient between Wheel/Road [-]"; J_FourWheels "Inertia Moment of four Wheels [kg m^2]"; Gravity "Gravity [m/s^2]"; Wheelbase "Wheelbase [m]"; COG_Height "Height Center of Gravity over Ground [m]"; COG_Front "Distance from Center of Gravity to Front Axle [m]"; COG_Rear "Distance from Center of Gravity to Rear Axle [m]"; Veh_Mass "Vehicle Mass [kg]"; LocalSampleTime "Local System Sample-Time [s]"
      mask help:
      | <Author> Alexander Koch, Benedikt Danquah based on Stefan Müller [1], Stephan Rohr [2]  </Author>
      | <Date> 15/01/2018 </Date>
      | <Sources>
      | [1] S. Mueller, S. Rohr, und et al, Hrsg, Analysing the Influence of Driver Behaviour and Tuning Measures on Battery Aging and Residual Value of Electric Vehicles, 2017
      | </Sources>
      |
      | <Description>
      | Calculates the longitudinal forces of the front and rear wheels, the rotational speed of the wheels and gives the roll resistant coefficient as an output. There are two roll resistant coefficients. A static parameter and a dynamic one. The dynamic roll resistant coefficient is mutliplied with the velocity and added to the static coefficient. Slip can not be represented. The moment of inertia is transfered to a mass.
      | </Description>
      mask init:
      | GlobalSampleTime = CalcGlobalSampleTime(LocalSampleTime);
      mask Help:
      | <Parameters>
      | Wheel Radius [m]
      | 	<Min> >0 </Min>
      | Roll Resistance Coefficient [-]
      | 	<Min> 0 </Min>
      | Dynamic Roll Resistance Coefficient [s/m]
      | Friction Coefficient between Wheel/Road [-]
      | Inertia Moment of four Wheels [kg m^2]
      | Gravity [m/s^2]
      | Wheelbase [m]
      | Height Center of Gravity over Ground [m]
      | Distance from Center of Gravity to Front Axle [m]
      | Distance from Center of Gravity to Rear Axle [m]
      | Local System Sample-Time [s]
      | 	<Min> GlobalSampleTime </Min>
      | Global Sample-Time [s]
      | </Parameters>
      | 
      | <Inputs>
      | FrontWheelsBrakeTrq [Nm]
      | 	 <sign orientation> [-] results in negative longitudinal driving Force </sign orientation>
      | RearWheelsBrakeTrq [Nm]
      | 	<sign orientation> [-] results in negative longitudinal driving Force </sign orientation>
      | FrontWheelsMotTrq [Nm]
      | 	<sign orientation> [+] results in positive longitudinal driving force </sign orientation>
      | RearWheelsMotTrq [Nm]
      | 	<sign orientation> [+] results in positive longitudinal driving force </sign orientation>
      | VehSpd [m/s]
      | VehAcc [m/s^2]
      | JRedIn [kg m^2]
      | GroundSlope [rad]
      | MassVehicle [kg]
      | </Inputs>
      | 
      | <Outputs>
      | FrontWheelsLongDriveForce [N]
      | RearWheelsLonDriveForce [N]
      | MaxTrqFrontWheels [Nm]
      | MaxTrqRearWheels [Nm]
      | WheelsRotSpd [rad/s]
      | RollResistCoeff [-]
      | MassJRed [kg]
      | </Outputs>
      | <Sources>
      | [1] S. Mueller, S. Rohr, W. Schmid, and M. Lienkamp, “Analysing the Influence of Driver Behaviour and Tuning Measures on Battery Aging and Residual Value of Electric Vehicles,” in Proc. EVS30 Symposium, Stuttgart, 2017, pp. 1–12.
      | [2] S. Rohr, “Technisch-wirtschaftliche Analyse des Zweitnutzungs- potentials von Lithium-Ionen-Traktionsbatterien,” Dissertation, Institute of Automotive Technology, Technical University Munich, Munich, 2018.
      | </Sources>
      mask TypeOptions Wheel_Radius: Wheel_Radius/Value
      mask TypeOptions Wheel_Roll_Resistance: Wheel_Roll_Resistance_Coeff/Value
      mask TypeOptions Wheel_Roll_Resistance_Dyn: Wheel_Roll_Resistance_Coeff_Dyn/Value
      mask TypeOptions mu_Tyre: mu_tyre/Value
      mask TypeOptions J_FourWheels: J_FourWheels/Value
      mask TypeOptions Gravity: Gravity/Value
      mask TypeOptions Wheelbase: Wheelbase/Value
      mask TypeOptions COG_Height: COG_Height/Value
      mask TypeOptions COG_Front: COG_Front/Value
      mask TypeOptions COG_Rear: COG_Rear/Value
      mask TypeOptions Veh_Mass: Vehicle_Mass/Value
      mask TypeOptions LocalSampleTime: FrontWheelsBrakeTrq [Nm]/SampleTime | RearWheelsBrakeTrq [Nm]/SampleTime | FrontWheelsMotTrq [Nm]/SampleTime | RearWheelsMotTrq [Nm]/SampleTime | VehSpd [m//s]/SampleTime | VehAcc [m//s^2]/SampleTime | JredIn [kg m^2]/SampleTime | GroundSlope [rad]/SampleTime
      mask DialogControl Container3 Prompt: Documentation
      mask DialogControl Control2 Prompt: %<MaskHelp>
      mask DialogControl Container5 Prompt: Sample Time
      mask Display:
      | [picturexpos,pictureypos,picturewidth,pictureheight] = ...
      |     CalcBlockPicturePosition(gcb,1,0.01,0.1,120,120); % calculating picture position depending on Block size and minimum margin size
      | image('Wheel_System_Const_R.svg',[picturexpos pictureypos picturewidth pictureheight]); % plot picture to block
  BUS_Out : Outport  VectorParamsAs1DForOutWhenUnconnected=off
  wires:
  BUS IN/1(BUS) -> BUS OUT/1(BUS)
  BUS_In/1 -> BUS IN/1(BUS_In)
  [TargetBrkTrqFront] -> Saturation/1
  [TargetBrkTrqRear] -> Saturation1/1
  BUS IN/5(TargetBrakeTrqFrontAxle [Nm]) -> [TargetBrkTrqFront]
  BUS IN/2(TargetDriveTrq [Nm]) -> Electric Drive Tabled Consumption/2(TargetTrq [Nm])  "TargetDriveTrq [Nm]"
  Electric Drive Tabled Consumption/1(DriveTrq [Nm]) -> Gear Stage/1, [DriveTrqEMotor]  "DriveTrq"
  Gear Stage/2 -> [OmegaEMOut]
  Constant/1 -> Wheel System Const R Const Coefficient/3(FrontWheelsMotTrq [Nm])
  [MomentofInertiaED] -> Gear Stage/3
  Gear Stage/1 -> [DriveWheelTrq], BUS OUT/3(In2)  "DriveWheelTorque [Nm]"
  [DriveWheelTrq] -> Wheel System Const R Const Coefficient/4(RearWheelsMotTrq [Nm])
  Gear Stage/3 -> [JredGearStage]
  [JredGearStage] -> Wheel System Const R Const Coefficient/7(JredIn [kg m^2])
  Wheel System Const R Const Coefficient/1(FrontWheelsLongDriveForce [N]) -> BUS OUT/4(In3)
  Wheel System Const R Const Coefficient/2(RearWheelsLongDriveForce [N]) -> BUS OUT/5(In4)
  Wheel System Const R Const Coefficient/3(MaxTrqRearWheels [Nm]) -> BUS OUT/6(In5)
  Wheel System Const R Const Coefficient/4(MaxTrqFrontWheels [Nm]) -> BUS OUT/7(In6)
  Wheel System Const R Const Coefficient/5(WheelsRotSpd [rad/s]) -> [WheelsRotSpeed], BUS OUT/8(In7)
  Wheel System Const R Const Coefficient/6(RollResistCoeff [-]) -> BUS OUT/9(In8)
  Wheel System Const R Const Coefficient/7(MassJRed [kg]) -> BUS OUT/10(In9)
  Electric Drive Tabled Consumption/2(DriveElectricPower [W]) -> UncertaintyTabledConsumption/1  "ElectricPower"
  Add2/1 -> [PowertrainPowerReq]  "PowertrainPowerReq"
  BUS IN/7(GroundSlope [rad]) -> Wheel System Const R Const Coefficient/8(GroundSlope [rad])
  Saturation/1 -> Wheel System Const R Const Coefficient/1(FrontWheelsBrakeTrq [Nm])
  Saturation1/1 -> Wheel System Const R Const Coefficient/2(RearWheelsBrakeTrq [Nm])
  [PowertrainPowerReq] -> BUS OUT/2(In1)  "PowertrainPowerReq [W]"
  [DrivePower] -> BUS OUT/11(In10)  "Drive Power [W]"
  [WheelsRotSpeed] -> Gear Stage/2
  [DriveTrqEMotor] -> BUS OUT/12(In11)  "DriveTrqEMotor [Nm]"
  [OmegaEMOut] -> BUS OUT/13(In12)  "OmegaEMOut [rad/s]"
  BUS IN/6(TargetBrakeTrqRearAxle [Nm]) -> [TargetBrkTrqRear]
  BUS IN/8(VehSpd [m/s]) -> [VehSpd]  "VehSpd [m/s]"
  [VehSpd] -> Wheel System Const R Const Coefficient/5(VehSpd [m/s])
  BUS IN/9(Acc [m/s^2]) -> [VehAcc]
  [VehAcc] -> Wheel System Const R Const Coefficient/6(VehAcc [m/s^2])
  [DriveTrqEMotor] -> Power Electronics Mapped Losses/2
  [OmegaEMOut] -> Power Electronics Mapped Losses/1
  Power Electronics Mapped Losses/1 -> UncertaintyMappedLosses/1
  [OmegaEMOut] -> Electric Drive Tabled Consumption/1(OmegaMot [rad/s])  "OmegaMot [rad/s]"
  Electric Drive Tabled Consumption/3(Momentofintertia [kg m^2]) -> [MomentofInertiaED]  "momentofinertia"
  BUS IN/3(MaxPower [W]) -> Electric Drive Tabled Consumption/3(MaxElectricPower [W])
  BUS IN/4(MinPower [W]) -> Electric Drive Tabled Consumption/4(MinElectricPower [W])
  BUS OUT/1(BUS_OUT) -> BUS_Out/1
  UncertaintyTabledConsumption/1 -> Add2/1, [DrivePower]
  UncertaintyMappedLosses/1 -> Add2/2
